simulink library "recursive_mean_lib"  (R2021a)
settings: Solver=VariableStepAuto  StartTime=0.0  StopTime=10.0  RelTol=1e-3
undefined symbols (not defined in the file or in its folder): DiscIntNeverNeededParam
settings Model: Creator=Rahul Subramanian  LastModifiedBy=Rahul Subramanian

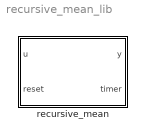
== system recursive_mean_lib ==
  recursive_mean : Subsystem

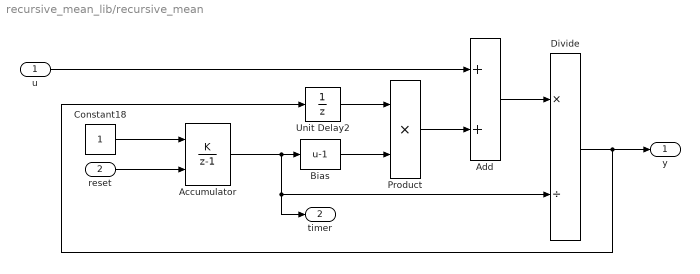
== system recursive_mean_lib/recursive_mean ==
  u : Inport
  reset : Inport  Port=2
  Accumulator : DiscreteIntegrator  IntegratorMethod=Accumulation: Forward Euler  ExternalReset=level  InitialCondition=1  SampleTime=-1  ICPrevOutput=DiscIntNeverNeededParam  ICPrevScaledInput=DiscIntNeverNeededParam
  Add : Sum
  Bias : Bias  Bias=-1
  Constant18 : Constant  OutDataTypeStr=Inherit: Inherit via back propagation
  Divide : Product  Inputs=*/
  Product : Product
  Unit Delay2 : UnitDelay  SampleTime=-1  HasFrameUpgradeWarning=on
  y : Outport
  timer : Outport  Port=2
  wires:
  Bias/1 -> Product/2
  Constant18/1 -> Accumulator/1
  Accumulator/1 -> timer/1, Divide/2, Bias/1
  Add/1 -> Divide/1
  Divide/1 -> y/1, Unit Delay2/1
  Unit Delay2/1 -> Product/1
  Product/1 -> Add/2
  u/1 -> Add/1
  reset/1 -> Accumulator/2
